simulink model "mrc"  (R2016b)
settings: Solver=ode45  StartTime=0.0  StopTime=inf  RelTol=1e-3  EnableMultiTasking=on
values from neighbouring files (symbols this model uses):
  amp_mp = [1 0.7 0.5]    [setup_mrc.m]    (also in sinal_para_vhdl.m)
  c = 3e8    (= 300000000)    [setup_mrc.m]    (also in sinal_para_vhdl.m)
  d = lambda/4    [setup_mrc.m]    (also in sinal_para_vhdl.m)
  dt = 1e-9    (= 1e-09)    [setup_mrc.m]    (also in sinal_para_vhdl.m = 1e-06)
  frequencia = 1e7    (= 10000000)    [setup_mrc.m]    (also in sinal_para_vhdl.m = 10000)
  tau_mp = [0 1e-7 1.5e-7]    [setup_mrc.m]    (also in sinal_para_vhdl.m = [0 1e-4 1.5e-4])
  theta_inc = [pi/20 pi/4 11*pi/6]    [setup_mrc.m]    (also in sinal_para_vhdl.m)
libraries: dsparch4 x4
settings Model: Creator=Leonardo  LastModifiedBy=root
settings DataIOCC: LimitDataPoints=on  SaveFormat=Array
settings OptimizationCC: LifeSpan=inf
settings DebuggingCC: SFUnexpectedBacktrackingDiag=warning  SFNoUnconditionalDefaultTransitionDiag=warning  SFExecutionAtInitializationDiag=none
settings HardwareCC: ProdBitPerPointer=32  ProdBitPerSizeT=32  ProdBitPerPtrDiffT=32  ProdLargestAtomicFloat=None  ProdIntDivRoundTo=Undefined  ProdEndianess=Unspecified  ProdWordSize=32  ProdHWDeviceType=32-bit Generic
settings ModelReferenceCC: PropagateSignalLabelsOutOfModel=off
settings GRTTargetCC: TargetLangStandard=C89/C90 (ANSI)  GeneratePreprocessorConditionals=Disable all
settings ConfigComp: CovMetricSettings=dw  CovHtmlReporting=on  CovSaveCumulativeToWorkspaceVar=on  CovSaveSingleToWorkspaceVar=on  CovExternalEMLEnable=off

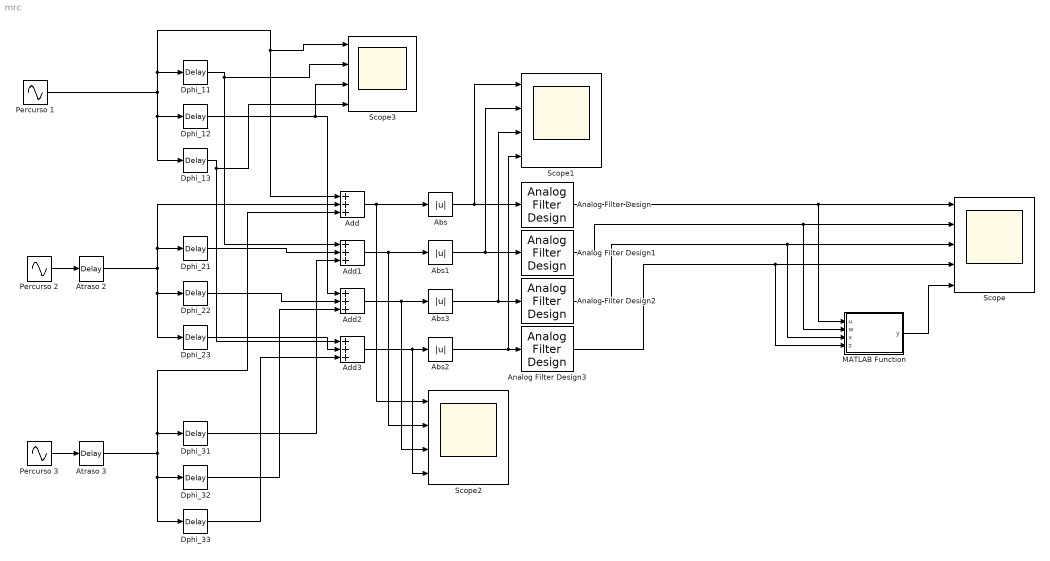
== system mrc ==
  Abs{,1..3} (4 alike) : Abs
  Add{,1..3} (4 alike) : Sum  Inputs=+++
  Analog Filter Design{,1..3} (4 alike) : dsparch4/Analog Filter Design  method=Butterworth  filttype=Lowpass  N=1  Wlo=2*pi*1000  Whi=80  Rp=2  Rs=40
  Atraso 2 : TransportDelay  DelayTime=tau_mp(2)
  Atraso 3 : TransportDelay  DelayTime=tau_mp(3)
  Dphi_11 : TransportDelay  DelayTime=(d/c)*sin(theta_inc(1))
  Dphi_12 : TransportDelay  DelayTime=2*(d/c)*sin(theta_inc(1))
  Dphi_13 : TransportDelay  DelayTime=3*(d/c)*sin(theta_inc(1))
  Dphi_21 : TransportDelay  DelayTime=(d/c)*sin(theta_inc(2))
  Dphi_22 : TransportDelay  DelayTime=2*(d/c)*sin(theta_inc(2))
  Dphi_23 : TransportDelay  DelayTime=3*(d/c)*sin(theta_inc(2))
  Dphi_31 : TransportDelay  DelayTime=(1/frequencia)+(d/c)*sin(theta_inc(3))
  Dphi_32 : TransportDelay  DelayTime=(1/frequencia)+2*(d/c)*sin(theta_inc(3))
  Dphi_33 : TransportDelay  DelayTime=(1/frequencia)+3*(d/c)*sin(theta_inc(3))
  MATLAB Function : MATLAB Function  TreatAsAtomicUnit=on
  Percurso 1 : Sin  Amplitude=amp_mp(1)  Frequency=2*pi*frequencia  Samples=100  SampleTime=dt
  Percurso 2 : Sin  Amplitude=amp_mp(2)  Frequency=2*pi*frequencia  Samples=100  SampleTime=dt
  Percurso 3 : Sin  Amplitude=amp_mp(3)  Frequency=2*pi*frequencia  Samples=100  SampleTime=dt
  Scope : Scope  NumInputPorts=5
  Scope1 : Scope  NumInputPorts=4
  Scope2 : Scope  NumInputPorts=4
  Scope3 : Scope  NumInputPorts=4
  wires:
  Percurso 2/1 -> Atraso 2/1
  Percurso 3/1 -> Atraso 3/1
  Percurso 1/1 -> Scope3/1, Add/1, Dphi_11/1, Dphi_13/1, Dphi_12/1
  Atraso 2/1 -> Add/2, Dphi_21/1, Dphi_23/1, Dphi_22/1
  Atraso 3/1 -> Add/3, Dphi_31/1, Dphi_33/1, Dphi_32/1
  Dphi_11/1 -> Scope3/2, Add1/1
  Dphi_21/1 -> Add1/2
  Dphi_31/1 -> Add1/3
  Dphi_12/1 -> Scope3/3, Add2/1
  Dphi_22/1 -> Add2/2
  Dphi_32/1 -> Add2/3
  Dphi_13/1 -> Scope3/4, Add3/1
  Dphi_23/1 -> Add3/2
  Dphi_33/1 -> Add3/3
  Add/1 -> Scope2/1, Abs/1
  Add1/1 -> Scope2/2, Abs1/1
  Add2/1 -> Scope2/3, Abs3/1
  Add3/1 -> Scope2/4, Abs2/1
  Abs/1 -> Scope1/1, Analog Filter Design/1
  Abs1/1 -> Scope1/2, Analog Filter Design1/1
  Abs2/1 -> Scope1/4, Analog Filter Design3/1
  Abs3/1 -> Scope1/3, Analog Filter Design2/1
  Analog Filter Design/1 -> MATLAB Function/1(u), Scope/1
  Analog Filter Design1/1 -> MATLAB Function/2(w), Scope/2
  Analog Filter Design2/1 -> MATLAB Function/3(x), Scope/3
  Analog Filter Design3/1 -> MATLAB Function/4(z), Scope/4
  MATLAB Function/1(y) -> Scope/5

== matlab function mrc/MATLAB Function ==
  data: u input; y output; w input; x input; z input
function y = fcn(u, w, x, z)

    if(u>w && u>x && u>z)
        y = u;
    elseif(w>u && w>x && w>z)
        y = w;
    elseif(x>u && x>w && x>z)
        y = x;
    elseif(z>u && z>w && z>x)
        y = z;
    else 
        y=u;
    end
